simulink model "regulator_LQG_discrete"  (R2021b)
settings: Solver=VariableStepAuto  StartTime=0.0  StopTime=10.0  RelTol=1e-3
values from neighbouring files (symbols this model uses):
  B_temp2 = [B ones(length(B),1)]    [main3.m]
  C_temp = eye(length(A))    [main3.m]
  D_temp2 = [D_temp zeros(length(D_temp),1)]    [main3.m]
  LQ_d = dlqr(A,B,Q,R)    [main3.m]
  R_tilde = 1    [main3.m]
  U_bar = Y_bar / G_1    [main3.m]
  x_0 = [5 20]'    [main3.m]
  X_bar = inv(eye(2)-A)*B*U_bar    [main3.m]
  Z = 0    [main3.m]
undefined symbols (not defined in the file or in its folder): A, B, C, D, Discrete, Time
libraries: simulink x2, ctrlSharedLib x1
settings Model: Creator=PaoloA  LastModifiedBy=PaoloA

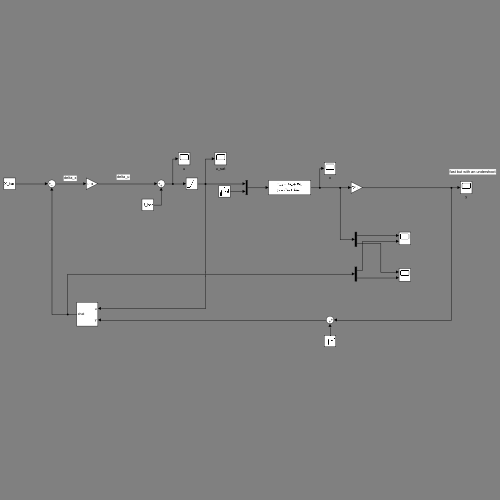
[thumbnail: Simulink's stored preview of the top-level diagram]
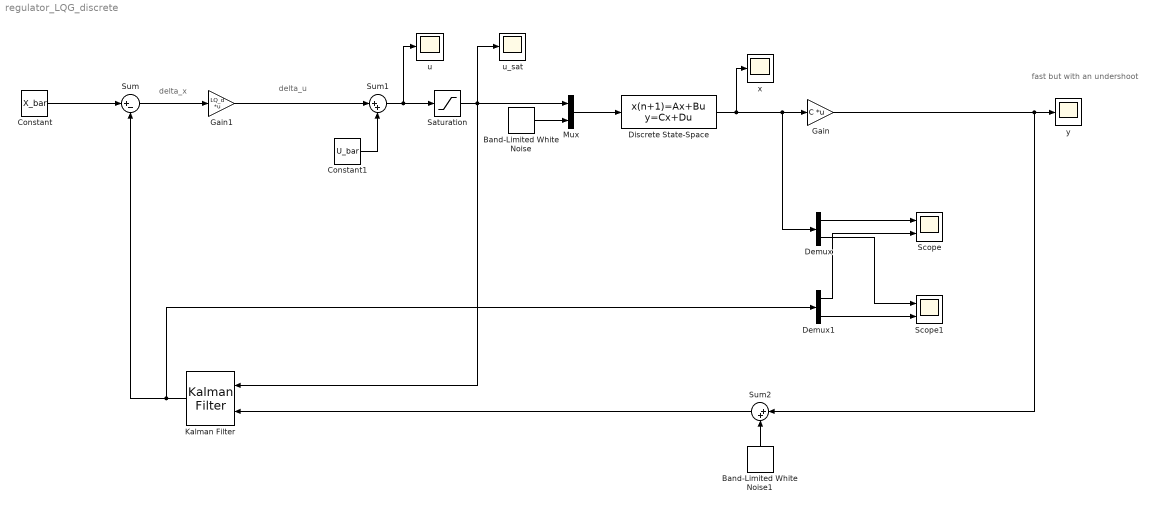
== system regulator_LQG_discrete ==
  note: delta_u
  note: delta_x
  note: fast but with an undershoot
  Band-Limited White Noise : simulink/Sources/Band-Limited White Noise  Cov=power_vx  Ts=0.1  seed=[23341]
  Band-Limited White Noise1 : simulink/Sources/Band-Limited White Noise  Cov=power_vy  Ts=0.1  seed=[23341]
  Constant : Constant  Value=X_bar
  Constant1 : Constant  Value=U_bar
  Demux : Demux  Outputs=2
  Demux1 : Demux  Outputs=2
  Discrete State-Space : DiscreteStateSpace  A=A  B=B_temp2  C=C_temp  D=D_temp2  InitialCondition=x_0  SampleTime=-1
  Gain : Gain  Gain=C  Multiplication=Matrix(K*u)
  Gain1 : Gain  Gain=LQ_d  Multiplication=Matrix(K*u)
  Kalman Filter : ctrlSharedLib/Kalman Filter  TimeDomain=Discrete-Time  UseCurrentEstimator=on  ModelSource=Individual A, B, C, D matrices  ModelSourceVariable=ss(0.95,1,1,0,1)  A=A  B=B  C=C  D=D  NumberOfStates=1  NumberOfInputs=1  NumberOfOutputs=1  InitialEstimateSource=Dialog  X0=0  P0=10  UseK=off  UseGH=off  NumberOfProcessNoiseInputs=1  G=1  TimeInvariantG=on  H=0  TimeInvariantH=on  Q=Q_tilde  TimeInvariantQ=on  R=R_tilde  TimeInvariantR=on  N=Z  TimeInvariantN=on  AddInputPort=on  AddEnablePort=off  OutputEstimatedY=off  OutputP=off  Ts=-1
  Mux : Mux  Inputs=2
  Saturation : Saturate  UpperLimit=+inf  LowerLimit=-inf
  Scope : Scope  NumInputPorts=2
  Scope1 : Scope  NumInputPorts=2
  Sum : Sum  Inputs=|+-
  Sum1 : Sum  Inputs=|++
  Sum2 : Sum  Inputs=|++
  u : Scope
  u_sat : Scope
  x : Scope
  y : Scope
  wires:
  Constant/1 -> Sum/1
  Saturation/1 -> Mux/1, u_sat/1, Kalman Filter/1
  Gain1/1 -> Sum1/1
  Gain/1 -> Sum2/1, y/1
  Discrete State-Space/1 -> x/1, Demux/1, Gain/1
  Sum1/1 -> u/1, Saturation/1
  Sum/1 -> Gain1/1
  Constant1/1 -> Sum1/2
  Kalman Filter/1 -> Demux1/1, Sum/2
  Mux/1 -> Discrete State-Space/1
  Band-Limited White Noise/1 -> Mux/2
  Demux/1 -> Scope/1
  Demux/2 -> Scope1/1
  Band-Limited White Noise1/1 -> Sum2/2
  Sum2/1 -> Kalman Filter/2
  Demux1/1 -> Scope/2
  Demux1/2 -> Scope1/2
